simulink model "BFE_TestHarness"  (Simulink 8.6)
settings: Solver=FixedStepDiscrete  StartTime=0.0  StopTime=3  FixedStep=Ts  RelTol=1e-3
PreLoadFcn:
  | addpath('MBD_Tests')
  | 
  | load('Workspace\EnvVar.mat')
  | run('MBD_Tests\MBD_tests_init.m')
  | if exist('tl_preloadfcn','file'), tl_preloadfcn(gcs,402); end
PostLoadFcn:
  | if exist('tl_postloadfcn','file'), tl_postloadfcn(gcs,402); end
InitFcn:
  | if exist('tlds_init','file'), tlds_init(gcs); end
StartFcn:
  | if exist('tlds_start','file'), tlds_start(gcs); end
StopFcn:
  | if exist('tlds_stop','file'), tlds_stop(gcs); end
undefined symbols (not defined in the file): ddv, Ts, u2, u3, u4
libraries: tllib x11, simulink x8, LIB_TF_G_111 x2, LIB_TF_G_12_StepControl x2, LIB_TF_G_112 x1, LIB_TF_G_113 x1
(part 1 of 17)
PreSaveFcn:
  | if exist('tl_presavefcn','file'), tl_presavefcn(gcs); end
CloseFcn:
  | if exist('tl_closefcn','file'), tl_closefcn(gcs); end
settings Model: TL_MAIN_DATA={'codeopt',{'linebreaklimit',150,'cleancode',1},'logopt',{'mdlrefmode',2},'date',737167.70554642356,'codegenerationmode',2}  TLRevision=402  DS_PROJECTFILE=BFE_Data.dd  Creator=cedric.sauvage  LastModifiedBy=pierre-olivier.pilot
settings DataIOCC: MaxDataPoints=16000  SignalLoggingSaveFormat=Dataset
settings OptimizationCC: BlockReduction=off  OptimizeBlockIOStorage=off  BufferReuse=off  GlobalBufferReuse=off  ExpressionFolding=off  LocalBlockOutputs=off
settings DebuggingCC: CheckSSInitialOutputMsg=off  FcnCallInpInsideContextMsg=UseLocalSettings  BusObjectLabelMismatch=error  StrictBusMsg=ErrorOnBusTreatedAsVector  NonBusSignalsTreatedAsBus=error
settings HardwareCC: ProdHWDeviceType=Generic->Unspecified (assume 32-bit Generic)
settings ModelReferenceCC: ModelReferenceNumInstancesAllowed=Single

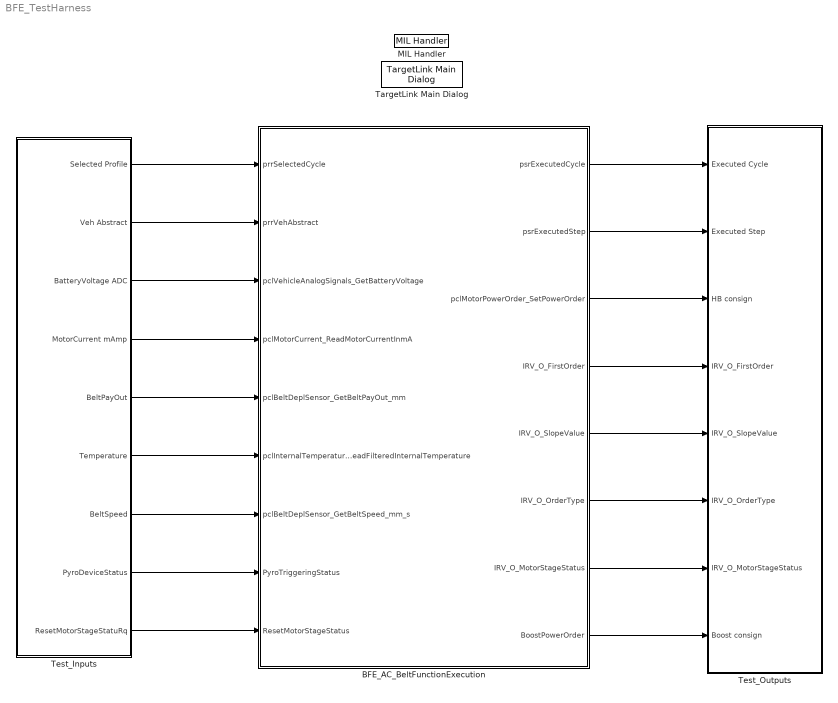
== system BFE_TestHarness ==
  BFE_AC_BeltFunctionExecution : Subsystem  Tag=TargetLink Simulation Frame  mask(TL_SimFrame){}
      settings: CopyFcn=if exist('tl_copyfcn','file'), tl_copyfcn(gcbh); end  NameChangeFcn=if exist('tl_framenamechangefcn','file'), tl_framenamechangefcn(gcbh); end
      settings: OpenFcn=|
      | if exist('open_tlsubsystem','file')
      |    open_tlsubsystem(gcbh);
      | else
      |    tlsubsystem = ...
      |       find_system(gcb, ...
      |       'LookUnderMasks','on', ...
      |       'FollowLinks','on', ...
      |       'Tag','MIL Subsystem');
      |    open_system(tlsubsystem);
      | end
      mask Display: disp('TargetLink\nModel-\nin-the-loop\nmode')
  MIL Handler : tllib/MIL Handler  data={'date',735951.66842159722}
  TargetLink Main Dialog : tllib/TargetLink Main Dialog  data=[]
  Test_Inputs : Subsystem
  Test_Outputs : Subsystem
  wires:
  Test_Inputs/2(Veh Abstract) -> BFE_AC_BeltFunctionExecution/2(prrVehAbstract)
  Test_Inputs/3(BatteryVoltage ADC) -> BFE_AC_BeltFunctionExecution/3(pclVehicleAnalogSignals_GetBatteryVoltage)
  Test_Inputs/4(MotorCurrent mAmp) -> BFE_AC_BeltFunctionExecution/4(pclMotorCurrent_ReadMotorCurrentInmA)
  Test_Inputs/5(BeltPayOut) -> BFE_AC_BeltFunctionExecution/5(pclBeltDeplSensor_GetBeltPayOut_mm)
  Test_Inputs/6(Temperature) -> BFE_AC_BeltFunctionExecution/6(pclInternalTemperature_ReadFilteredInternalTemperature)
  Test_Inputs/7(BeltSpeed) -> BFE_AC_BeltFunctionExecution/7(pclBeltDeplSensor_GetBeltSpeed_mm_s)
  Test_Inputs/1(Selected Profile) -> BFE_AC_BeltFunctionExecution/1(prrSelectedCycle)
  BFE_AC_BeltFunctionExecution/1(psrExecutedCycle) -> Test_Outputs/1(Executed Cycle)
  BFE_AC_BeltFunctionExecution/2(psrExecutedStep) -> Test_Outputs/2(Executed Step)
  BFE_AC_BeltFunctionExecution/3(pclMotorPowerOrder_SetPowerOrder) -> Test_Outputs/3(HB consign)
  Test_Inputs/8(PyroDeviceStatus) -> BFE_AC_BeltFunctionExecution/8(PyroTriggeringStatus)
  BFE_AC_BeltFunctionExecution/4(IRV_O_FirstOrder) -> Test_Outputs/4(IRV_O_FirstOrder)
  BFE_AC_BeltFunctionExecution/5(IRV_O_SlopeValue) -> Test_Outputs/5(IRV_O_SlopeValue)
  BFE_AC_BeltFunctionExecution/6(IRV_O_OrderType) -> Test_Outputs/6(IRV_O_OrderType)
  BFE_AC_BeltFunctionExecution/7(IRV_O_MotorStageStatus) -> Test_Outputs/7(IRV_O_MotorStageStatus)
  BFE_AC_BeltFunctionExecution/8(BoostPowerOrder) -> Test_Outputs/8(Boost consign)
  Test_Inputs/9(ResetMotorStageStatuRq) -> BFE_AC_BeltFunctionExecution/9(ResetMotorStageStatus)

== system BFE_TestHarness/BFE_AC_BeltFunctionExecution ==
  prrSelectedCycle : Inport
  prrVehAbstract : Inport  Port=2
  pclVehicleAnalogSignals_GetBatteryVoltage : Inport  Port=3
  pclMotorCurrent_ReadMotorCurrentInmA : Inport  Port=4
  pclBeltDeplSensor_GetBeltPayOut_mm : Inport  Port=5
  pclInternalTemperature_ReadFilteredInternalTemperature : Inport  Port=6
  pclBeltDeplSensor_GetBeltSpeed_mm_s : Inport  Port=7
  PyroTriggeringStatus : Inport  Port=8
  ResetMotorStageStatus : Inport  Port=9
  Subsystem : Subsystem  Tag=struct('sfcnName','BFE_AC_BeltFunctionExecution_sf','subFunction','','srcSubsystem','')  mask(TL_Enable){}
      settings: OpenFcn=warndlg(get_param(gcb,'MaskHelp'),'Serious Warning');
      mask Help: This subsystem keeps the TargetLink subsystem (subsystem with TargetLink blocks for production code generation), and is needed for the TargetLink simulation frame to work properly. DO NOT DELETE OR MODIFY IT!
  psrExecutedCycle : Outport
  psrExecutedStep : Outport  Port=2
  pclMotorPowerOrder_SetPowerOrder : Outport  Port=3
  IRV_O_FirstOrder : Outport  Port=4
  IRV_O_SlopeValue : Outport  Port=5
  IRV_O_OrderType : Outport  Port=6
  IRV_O_MotorStageStatus : Outport  Port=7
  BoostPowerOrder : Outport  Port=8
  wires:
  prrSelectedCycle/1 -> Subsystem/1(prrSelectedCycle)
  prrVehAbstract/1 -> Subsystem/2(prrVehAbstract)
  pclVehicleAnalogSignals_GetBatteryVoltage/1 -> Subsystem/3(pclVehicleAnalogSignals_GetBatteryVoltage)
  pclMotorCurrent_ReadMotorCurrentInmA/1 -> Subsystem/4(pclMotorCurrent_ReadMotorCurrentInmA)
  pclBeltDeplSensor_GetBeltPayOut_mm/1 -> Subsystem/5(pclBeltDeplSensor_GetBeltPayOut_mm)
  pclInternalTemperature_ReadFilteredInternalTemperature/1 -> Subsystem/6(pclInternalTemperature_ReadFilteredInternalTemperature)
  pclBeltDeplSensor_GetBeltSpeed_mm_s/1 -> Subsystem/7(pclBeltDeplSensor_GetBeltSpeed_mm_s)
  PyroTriggeringStatus/1 -> Subsystem/8(PyroTriggeringStatus)
  ResetMotorStageStatus/1 -> Subsystem/9(ResetMotorStageStatus)
  Subsystem/1(psrExecutedCycle) -> psrExecutedCycle/1
  Subsystem/2(psrExecutedStep) -> psrExecutedStep/1
  Subsystem/3(pclMotorPowerOrder_SetPowerOrder) -> pclMotorPowerOrder_SetPowerOrder/1
  Subsystem/4(IRV_O_FirstOrder) -> IRV_O_FirstOrder/1
  Subsystem/5(IRV_O_SlopeValue) -> IRV_O_SlopeValue/1
  Subsystem/6(IRV_O_OrderType) -> IRV_O_OrderType/1
  Subsystem/7(IRV_O_MotorStageStatus) -> IRV_O_MotorStageStatus/1
  Subsystem/8(BoostPowerOrder) -> BoostPowerOrder/1

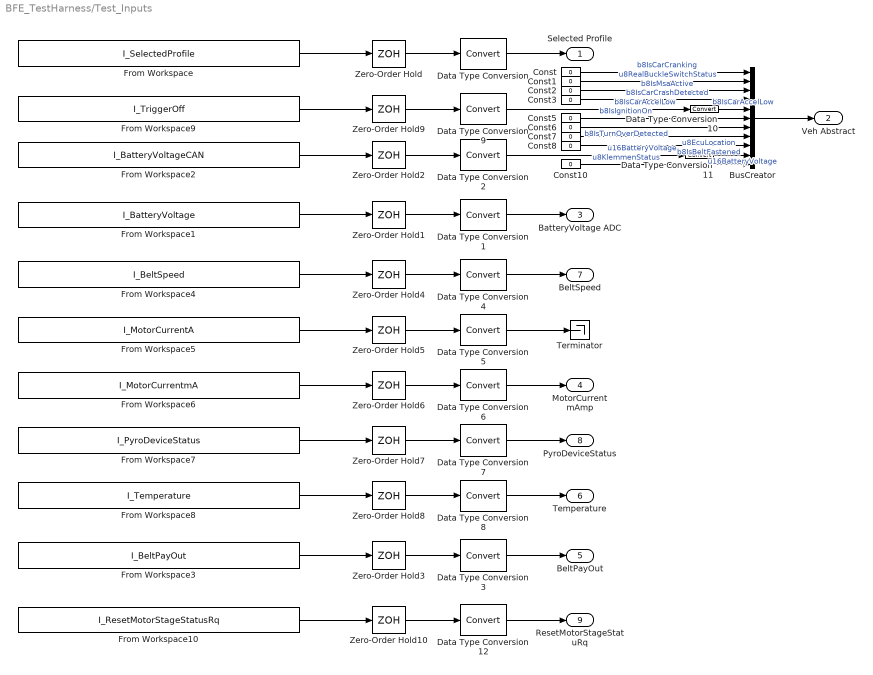
== system BFE_TestHarness/Test_Inputs ==
  BusCreator : BusCreator  Inputs=11
  Const{,1..3,5..8,10} (9 alike) : Constant  Value=0
  Data Type Conversion{,1..12} (13 alike) : DataTypeConversion
  From Workspace : FromWorkspace  VariableName=I_SelectedProfile  SampleTime=Ts  OutputAfterFinalValue=Holding final value
  From Workspace1 : FromWorkspace  VariableName=I_BatteryVoltage  SampleTime=Ts
  From Workspace10 : FromWorkspace  VariableName=I_ResetMotorStageStatusRq  SampleTime=Ts
  From Workspace2 : FromWorkspace  VariableName=I_BatteryVoltageCAN  SampleTime=Ts
  From Workspace3 : FromWorkspace  VariableName=I_BeltPayOut  SampleTime=Ts
  From Workspace4 : FromWorkspace  VariableName=I_BeltSpeed  SampleTime=Ts
  From Workspace5 : FromWorkspace  VariableName=I_MotorCurrentA  SampleTime=Ts
  From Workspace6 : FromWorkspace  VariableName=I_MotorCurrentmA  SampleTime=Ts
  From Workspace7 : FromWorkspace  VariableName=I_PyroDeviceStatus  SampleTime=Ts
  From Workspace8 : FromWorkspace  VariableName=I_Temperature  SampleTime=Ts
  From Workspace9 : FromWorkspace  VariableName=I_TriggerOff  SampleTime=Ts
  Terminator : Terminator
  Zero-Order Hold : ZeroOrderHold  SampleTime=-1
  Zero-Order Hold{1..10} (10 alike) : ZeroOrderHold  SampleTime=Ts
  Selected Profile : Outport
  Veh Abstract : Outport  Port=2
  BatteryVoltage ADC : Outport  Port=3
  MotorCurrent mAmp : Outport  Port=4
  BeltPayOut : Outport  Port=5
  Temperature : Outport  Port=6
  BeltSpeed : Outport  Port=7
  PyroDeviceStatus : Outport  Port=8
  ResetMotorStageStatuRq : Outport  Port=9
  wires:
  From Workspace/1 -> Zero-Order Hold/1
  Data Type Conversion/1 -> Selected Profile/1
  Zero-Order Hold1/1 -> Data Type Conversion1/1
  Data Type Conversion1/1 -> BatteryVoltage ADC/1
  Zero-Order Hold2/1 -> Data Type Conversion2/1
  Data Type Conversion2/1 -> Data Type Conversion11/1  "u16BatteryVoltage"
  Zero-Order Hold3/1 -> Data Type Conversion3/1
  Data Type Conversion3/1 -> BeltPayOut/1
  Zero-Order Hold4/1 -> Data Type Conversion4/1
  Data Type Conversion4/1 -> BeltSpeed/1
  Zero-Order Hold5/1 -> Data Type Conversion5/1
  Data Type Conversion5/1 -> Terminator/1
  Zero-Order Hold6/1 -> Data Type Conversion6/1
  Data Type Conversion6/1 -> MotorCurrent mAmp/1
  Zero-Order Hold7/1 -> Data Type Conversion7/1
  Data Type Conversion7/1 -> PyroDeviceStatus/1
  Zero-Order Hold8/1 -> Data Type Conversion8/1
  Data Type Conversion8/1 -> Temperature/1
  Zero-Order Hold9/1 -> Data Type Conversion9/1
  Data Type Conversion9/1 -> Data Type Conversion10/1  "b8IsCarAccelLow"
  From Workspace1/1 -> Zero-Order Hold1/1
  From Workspace2/1 -> Zero-Order Hold2/1
  From Workspace3/1 -> Zero-Order Hold3/1
  From Workspace4/1 -> Zero-Order Hold4/1
  From Workspace5/1 -> Zero-Order Hold5/1
  From Workspace6/1 -> Zero-Order Hold6/1
  From Workspace7/1 -> Zero-Order Hold7/1
  From Workspace8/1 -> Zero-Order Hold8/1
  From Workspace9/1 -> Zero-Order Hold9/1
  Const/1 -> BusCreator/1  "b8IsCarCranking"
  Const1/1 -> BusCreator/2  "u8RealBuckleSwitchStatus"
  Const2/1 -> BusCreator/3  "b8IsMsaActive"
  Const3/1 -> BusCreator/4  "b8IsCarCrashDetected"
  Const5/1 -> BusCreator/6  "b8IsIgnitionOn"
  Const6/1 -> BusCreator/7  "b8IsTurnOverDetected"
  Const7/1 -> BusCreator/8  "u8EcuLocation"
  Const8/1 -> BusCreator/9  "b8IsBeltFastened"
  Const10/1 -> BusCreator/11  "u8KlemmenStatus"
  Data Type Conversion10/1 -> BusCreator/5  "b8IsCarAccelLow"
  Data Type Conversion11/1 -> BusCreator/10  "u16BatteryVoltage"
  BusCreator/1 -> Veh Abstract/1
  Zero-Order Hold/1 -> Data Type Conversion/1
  Zero-Order Hold10/1 -> Data Type Conversion12/1
  Data Type Conversion12/1 -> ResetMotorStageStatuRq/1
  From Workspace10/1 -> Zero-Order Hold10/1

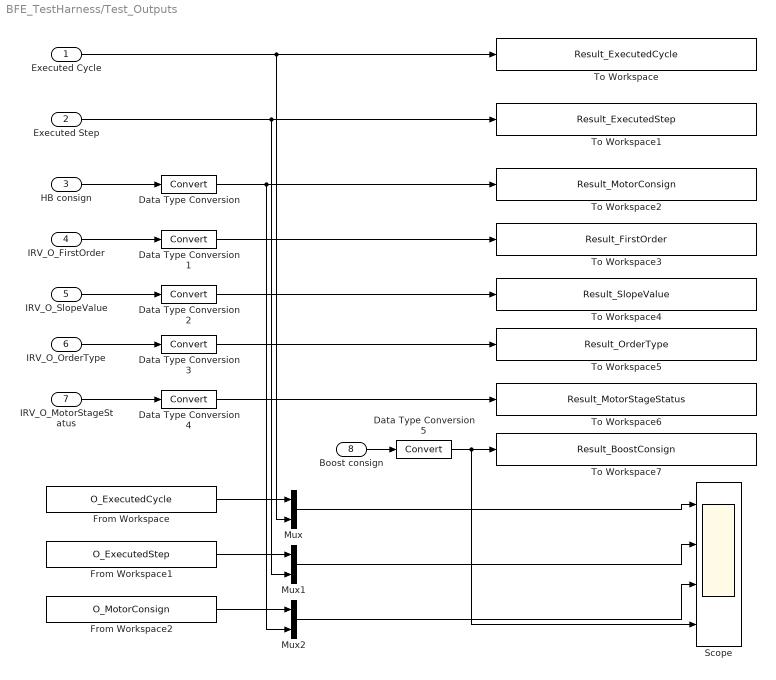
== system BFE_TestHarness/Test_Outputs ==
  Executed Cycle : Inport
  Executed Step : Inport  Port=2
  HB consign : Inport  Port=3
  IRV_O_FirstOrder : Inport  Port=4
  IRV_O_SlopeValue : Inport  Port=5
  IRV_O_OrderType : Inport  Port=6
  IRV_O_MotorStageStatus : Inport  Port=7
  Boost consign : Inport  Port=8
  Data Type Conversion{,1..5} (6 alike) : DataTypeConversion
  From Workspace : FromWorkspace  VariableName=O_ExecutedCycle  SampleTime=Ts
  From Workspace1 : FromWorkspace  VariableName=O_ExecutedStep  SampleTime=Ts
  From Workspace2 : FromWorkspace  VariableName=O_MotorConsign  SampleTime=Ts
  Mux : Mux  Inputs=2
  Mux1 : Mux  Inputs=2
  Mux2 : Mux  Inputs=2
  Scope : Scope  NumInputPorts=4
  To Workspace : ToWorkspace  VariableName=Result_ExecutedCycle  SaveFormat=Structure With Time  SampleTime=-1
  To Workspace1 : ToWorkspace  VariableName=Result_ExecutedStep  SaveFormat=Structure  SampleTime=-1
  To Workspace2 : ToWorkspace  VariableName=Result_MotorConsign  SaveFormat=Structure  SampleTime=-1
  To Workspace3 : ToWorkspace  VariableName=Result_FirstOrder  SaveFormat=Structure  SampleTime=-1
  To Workspace4 : ToWorkspace  VariableName=Result_SlopeValue  SaveFormat=Structure  SampleTime=-1
  To Workspace5 : ToWorkspace  VariableName=Result_OrderType  SaveFormat=Structure  SampleTime=-1
  To Workspace6 : ToWorkspace  VariableName=Result_MotorStageStatus  SaveFormat=Structure  SampleTime=-1
  To Workspace7 : ToWorkspace  VariableName=Result_BoostConsign  SaveFormat=Structure  SampleTime=-1
  wires:
  Executed Cycle/1 -> To Workspace/1, Mux/2
  Executed Step/1 -> To Workspace1/1, Mux1/2
  HB consign/1 -> Data Type Conversion/1
  Mux/1 -> Scope/1
  Mux1/1 -> Scope/2
  Mux2/1 -> Scope/3
  From Workspace/1 -> Mux/1
  From Workspace1/1 -> Mux1/1
  From Workspace2/1 -> Mux2/1
  Data Type Conversion/1 -> To Workspace2/1, Mux2/2
  IRV_O_FirstOrder/1 -> Data Type Conversion1/1
  IRV_O_SlopeValue/1 -> Data Type Conversion2/1
  IRV_O_OrderType/1 -> Data Type Conversion3/1
  Data Type Conversion1/1 -> To Workspace3/1
  Data Type Conversion2/1 -> To Workspace4/1
  Data Type Conversion3/1 -> To Workspace5/1
  IRV_O_MotorStageStatus/1 -> Data Type Conversion4/1
  Data Type Conversion4/1 -> To Workspace6/1
  Boost consign/1 -> Data Type Conversion5/1
  Data Type Conversion5/1 -> To Workspace7/1, Scope/4

== system BFE_TestHarness/BFE_AC_BeltFunctionExecution/Subsystem ==
  prrSelectedCycle : Inport
  prrVehAbstract : Inport  Port=2
  pclVehicleAnalogSignals_GetBatteryVoltage : Inport  Port=3
  pclMotorCurrent_ReadMotorCurrentInmA : Inport  Port=4
  pclBeltDeplSensor_GetBeltPayOut_mm : Inport  Port=5
  pclInternalTemperature_ReadFilteredInternalTemperature : Inport  Port=6
  pclBeltDeplSensor_GetBeltSpeed_mm_s : Inport  Port=7
  PyroTriggeringStatus : Inport  Port=8
  ResetMotorStageStatus : Inport  Port=9
  BFE_AC_BeltFunctionExecution : Subsystem  Tag=MIL Subsystem  Description=a  mask(MIL Subsystem){}
      settings: CopyFcn=if exist('tl_copyfcn','file'), tl_copyfcn(gcbh); end  NameChangeFcn=if exist('tl_namechangefcn','file'), tl_namechangefcn(gcbh); end  DestroyFcn=if exist('update_tl_main_dlg','file'), update_tl_main_dlg('TL_subs_display'); end
      mask Display: disp('TargetLink Subsystem')
  psrExecutedCycle : Outport
  psrExecutedStep : Outport  Port=2
  pclMotorPowerOrder_SetPowerOrder : Outport  Port=3
  IRV_O_FirstOrder : Outport  Port=4
  IRV_O_SlopeValue : Outport  Port=5
  IRV_O_OrderType : Outport  Port=6
  IRV_O_MotorStageStatus : Outport  Port=7
  BoostPowerOrder : Outport  Port=8
  wires:
  prrSelectedCycle/1 -> BFE_AC_BeltFunctionExecution/1(prrSelectedCycle)
  prrVehAbstract/1 -> BFE_AC_BeltFunctionExecution/2(prrVehAbstract)
  pclVehicleAnalogSignals_GetBatteryVoltage/1 -> BFE_AC_BeltFunctionExecution/3(pclVehicleAnalogSignals_GetBatteryVoltage)
  pclMotorCurrent_ReadMotorCurrentInmA/1 -> BFE_AC_BeltFunctionExecution/4(pclMotorCurrent_ReadMotorCurrentInmA)
  pclBeltDeplSensor_GetBeltPayOut_mm/1 -> BFE_AC_BeltFunctionExecution/5(pclBeltDeplSensor_GetBeltPayOut_mm)
  pclInternalTemperature_ReadFilteredInternalTemperature/1 -> BFE_AC_BeltFunctionExecution/6(pclInternalTemperature_ReadFilteredInternalTemperature)
  pclBeltDeplSensor_GetBeltSpeed_mm_s/1 -> BFE_AC_BeltFunctionExecution/7(pclBeltDeplSensor_GetBeltSpeed_mm_s)
  PyroTriggeringStatus/1 -> BFE_AC_BeltFunctionExecution/8(PyroTriggeringStatus)
  ResetMotorStageStatus/1 -> BFE_AC_BeltFunctionExecution/9(ResetMotorStageStatus)
  BFE_AC_BeltFunctionExecution/1(psrExecutedCycle) -> psrExecutedCycle/1
  BFE_AC_BeltFunctionExecution/2(psrExecutedStep) -> psrExecutedStep/1
  BFE_AC_BeltFunctionExecution/3(pclMotorPowerOrder_SetPowerOrder) -> pclMotorPowerOrder_SetPowerOrder/1
  BFE_AC_BeltFunctionExecution/4(IRV_O_FirstOrder) -> IRV_O_FirstOrder/1
  BFE_AC_BeltFunctionExecution/5(IRV_O_SlopeValue) -> IRV_O_SlopeValue/1
  BFE_AC_BeltFunctionExecution/6(IRV_O_OrderType) -> IRV_O_OrderType/1
  BFE_AC_BeltFunctionExecution/7(IRV_O_MotorStageStatus) -> IRV_O_MotorStageStatus/1
  BFE_AC_BeltFunctionExecution/8(BoostPowerOrder) -> BoostPowerOrder/1

== system BFE_TestHarness/BFE_AC_BeltFunctionExecution/Subsystem/BFE_AC_BeltFunctionExecution ==
  prrSelectedCycle : Inport
      settings: NameChangeFcn=if exist('tl_check_ports','file'), tl_check_ports(gcbh); end
      settings: CopyFcn=|
      | if exist('tl_reset_reviewflag','file')==2
      |     tl_reset_reviewflag(gcbh);
      | end
      | if exist('tl_check_ports','file')
      |     tl_check_ports(gcbh);
      | end
  prrVehAbstract : Inport  Port=2
      settings: NameChangeFcn=if exist('tl_check_ports','file'), tl_check_ports(gcbh); end
      settings: CopyFcn=|
      | if exist('tl_reset_reviewflag','file')==2
      |     tl_reset_reviewflag(gcbh);
      | end
      | if exist('tl_check_ports','file')
      |     tl_check_ports(gcbh);
      | end
  pclVehicleAnalogSignals_GetBatteryVoltage : Inport  Port=3
      settings: NameChangeFcn=if exist('tl_check_ports','file'), tl_check_ports(gcbh); end
      settings: CopyFcn=|
      | if exist('tl_reset_reviewflag','file')==2
      |     tl_reset_reviewflag(gcbh);
      | end
      | if exist('tl_check_ports','file')
      |     tl_check_ports(gcbh);
      | end
  pclMotorCurrent_ReadMotorCurrentInmA : Inport  Port=4
      settings: NameChangeFcn=if exist('tl_check_ports','file'), tl_check_ports(gcbh); end
      settings: CopyFcn=|
      | if exist('tl_reset_reviewflag','file')==2
      |     tl_reset_reviewflag(gcbh);
      | end
      | if exist('tl_check_ports','file')
      |     tl_check_ports(gcbh);
      | end
  pclBeltDeplSensor_GetBeltPayOut_mm : Inport  Port=5
      settings: NameChangeFcn=if exist('tl_check_ports','file'), tl_check_ports(gcbh); end
      settings: CopyFcn=|
      | if exist('tl_reset_reviewflag','file')==2
      |     tl_reset_reviewflag(gcbh);
      | end
      | if exist('tl_check_ports','file')
      |     tl_check_ports(gcbh);
      | end
  pclInternalTemperature_ReadFilteredInternalTemperature : Inport  Port=6
      settings: NameChangeFcn=if exist('tl_check_ports','file'), tl_check_ports(gcbh); end
      settings: CopyFcn=|
      | if exist('tl_reset_reviewflag','file')==2
      |     tl_reset_reviewflag(gcbh);
      | end
      | if exist('tl_check_ports','file')
      |     tl_check_ports(gcbh);
      | end
  pclBeltDeplSensor_GetBeltSpeed_mm_s : Inport  Port=7
      settings: NameChangeFcn=if exist('tl_check_ports','file'), tl_check_ports(gcbh); end
      settings: CopyFcn=|
      | if exist('tl_reset_reviewflag','file')==2
      |     tl_reset_reviewflag(gcbh);
      | end
      | if exist('tl_check_ports','file')
      |     tl_check_ports(gcbh);
      | end
  PyroTriggeringStatus : Inport  Port=8  mask(TL_Inport){data={'output',{'type','UInt8'},'date',735951.6686239352}}
      settings: DeleteFcn=if exist('delete_tlblock','file')==2,delete_tlblock(gcbh);end  OpenFcn=if exist('tl_open_blockdlg','file')==2,tl_open_blockdlg(gcbh);else,open_system(gcbh,'parameter');end
      settings: CopyFcn=|
      | if exist('tl_reset_reviewflag','file')==2
      |     tl_reset_reviewflag(gcbh);
      | end
      | if exist('tl_check_ports','file')
      |     tl_check_ports(gcbh);
      | end
      settings: NameChangeFcn=|
      | if exist('rename_tlblock','file')==2,rename_tlblock(gcbh);end
      | if exist('tl_check_ports','file'), tl_check_ports(gcbh); end
      mask Help: eval(['if exist(''tl_online_help'',''file'') == 2, tl_online_help(''Topic'',''TL_Inport''),else, web([''jar:file:///'',matlabroot,''/help/toolbox/simulink/help.jar!/slref/' lower(get_param(gcbh,'Blocktype')) '.html''], ''-helpbrowser''),end'])
      mask Display: plot([0.2 0.35 NaN 0.65 0.8],[0 1 NaN 0 1]);
  ResetMotorStageStatus : Inport  Port=9  mask(TL_Inport){data={'output',{'type','UInt8'},'date',735951.6686239352}}
      settings: DeleteFcn=if exist('delete_tlblock','file')==2,delete_tlblock(gcbh);end  OpenFcn=if exist('tl_open_blockdlg','file')==2,tl_open_blockdlg(gcbh);else,open_system(gcbh,'parameter');end
      settings: CopyFcn=|
      | if exist('tl_reset_reviewflag','file')==2
      |     tl_reset_reviewflag(gcbh);
      | end
      | if exist('tl_check_ports','file')
      |     tl_check_ports(gcbh);
      | end
      settings: NameChangeFcn=|
      | if exist('rename_tlblock','file')==2,rename_tlblock(gcbh);end
      | if exist('tl_check_ports','file'), tl_check_ports(gcbh); end
      mask Help: eval(['if exist(''tl_online_help'',''file'') == 2, tl_online_help(''Topic'',''TL_Inport''),else, web([''jar:file:///'',matlabroot,''/help/toolbox/simulink/help.jar!/slref/' lower(get_param(gcbh,'Blocktype')) '.html''], ''-helpbrowser''),end'])
      mask Display: plot([0.2 0.35 NaN 0.65 0.8],[0 1 NaN 0 1]);
  BFE_AC_BeltFunctionExecution : Subsystem
  psrExecutedCycle : Outport
      settings: NameChangeFcn=if exist('tl_check_ports','file'), tl_check_ports(gcbh); end
      settings: CopyFcn=|
      | if exist('tl_reset_reviewflag','file')==2
      |     tl_reset_reviewflag(gcbh);
      | end
      | if exist('tl_check_ports','file')
      |     tl_check_ports(gcbh);
      | end
  psrExecutedStep : Outport  Port=2
      settings: NameChangeFcn=if exist('tl_check_ports','file'), tl_check_ports(gcbh); end
      settings: CopyFcn=|
      | if exist('tl_reset_reviewflag','file')==2
      |     tl_reset_reviewflag(gcbh);
      | end
      | if exist('tl_check_ports','file')
      |     tl_check_ports(gcbh);
      | end
  pclMotorPowerOrder_SetPowerOrder : Outport  Port=3  mask(TL_Outport){data={'date',735951.66842629632}}
      settings: DeleteFcn=if exist('delete_tlblock','file')==2,delete_tlblock(gcbh);end  OpenFcn=if exist('tl_open_blockdlg','file')==2,tl_open_blockdlg(gcbh);else,open_system(gcbh,'parameter');end
      settings: CopyFcn=|
      | if exist('tl_reset_reviewflag','file')==2
      |     tl_reset_reviewflag(gcbh);
      | end
      | if exist('tl_check_ports','file')
      |     tl_check_ports(gcbh);
      | end
      settings: NameChangeFcn=|
      | if exist('rename_tlblock','file')==2,rename_tlblock(gcbh);end
      | if exist('tl_check_ports','file'), tl_check_ports(gcbh); end
      mask Help: eval(['if exist(''tl_online_help'',''file'') == 2, tl_online_help(''Topic'',''TL_Outport''),else, web([''jar:file:///'',matlabroot,''/help/toolbox/simulink/help.jar!/slref/' lower(get_param(gcbh,'Blocktype')) '.html''], ''-helpbrowser''),end'])
      mask Display: plot([0.2 0.35 NaN 0.65 0.8],[0 1 NaN 0 1]);
  IRV_O_FirstOrder : Outport  Port=4  mask(TL_Outport){data={'output',{'type','Int32'},'date',735951.66842549772}}
      settings: DeleteFcn=if exist('delete_tlblock','file')==2,delete_tlblock(gcbh);end  OpenFcn=if exist('tl_open_blockdlg','file')==2,tl_open_blockdlg(gcbh);else,open_system(gcbh,'parameter');end
      settings: CopyFcn=|
      | if exist('tl_reset_reviewflag','file')==2
      |     tl_reset_reviewflag(gcbh);
      | end
      | if exist('tl_check_ports','file')
      |     tl_check_ports(gcbh);
      | end
      settings: NameChangeFcn=|
      | if exist('rename_tlblock','file')==2,rename_tlblock(gcbh);end
      | if exist('tl_check_ports','file'), tl_check_ports(gcbh); end
      mask Help: eval(['if exist(''tl_online_help'',''file'') == 2, tl_online_help(''Topic'',''TL_Outport''),else, web([''jar:file:///'',matlabroot,''/help/toolbox/simulink/help.jar!/slref/' lower(get_param(gcbh,'Blocktype')) '.html''], ''-helpbrowser''),end'])
      mask Display: plot([0.2 0.35 NaN 0.65 0.8],[0 1 NaN 0 1]);
  IRV_O_SlopeValue : Outport  Port=5  mask(TL_Outport){data={'output',{'type','Int32'},'date',735951.66842468746}}
      settings: DeleteFcn=if exist('delete_tlblock','file')==2,delete_tlblock(gcbh);end  OpenFcn=if exist('tl_open_blockdlg','file')==2,tl_open_blockdlg(gcbh);else,open_system(gcbh,'parameter');end
      settings: CopyFcn=|
      | if exist('tl_reset_reviewflag','file')==2
      |     tl_reset_reviewflag(gcbh);
      | end
      | if exist('tl_check_ports','file')
      |     tl_check_ports(gcbh);
      | end
      settings: NameChangeFcn=|
      | if exist('rename_tlblock','file')==2,rename_tlblock(gcbh);end
      | if exist('tl_check_ports','file'), tl_check_ports(gcbh); end
      mask Help: eval(['if exist(''tl_online_help'',''file'') == 2, tl_online_help(''Topic'',''TL_Outport''),else, web([''jar:file:///'',matlabroot,''/help/toolbox/simulink/help.jar!/slref/' lower(get_param(gcbh,'Blocktype')) '.html''], ''-helpbrowser''),end'])
      mask Display: plot([0.2 0.35 NaN 0.65 0.8],[0 1 NaN 0 1]);
  IRV_O_OrderType : Outport  Port=6  mask(TL_Outport){data={'output',{'type','UInt8'},'date',735951.66842387733}}
      settings: DeleteFcn=if exist('delete_tlblock','file')==2,delete_tlblock(gcbh);end  OpenFcn=if exist('tl_open_blockdlg','file')==2,tl_open_blockdlg(gcbh);else,open_system(gcbh,'parameter');end
      settings: CopyFcn=|
      | if exist('tl_reset_reviewflag','file')==2
      |     tl_reset_reviewflag(gcbh);
      | end
      | if exist('tl_check_ports','file')
      |     tl_check_ports(gcbh);
      | end
      settings: NameChangeFcn=|
      | if exist('rename_tlblock','file')==2,rename_tlblock(gcbh);end
      | if exist('tl_check_ports','file'), tl_check_ports(gcbh); end
      mask Help: eval(['if exist(''tl_online_help'',''file'') == 2, tl_online_help(''Topic'',''TL_Outport''),else, web([''jar:file:///'',matlabroot,''/help/toolbox/simulink/help.jar!/slref/' lower(get_param(gcbh,'Blocktype')) '.html''], ''-helpbrowser''),end'])
      mask Display: plot([0.2 0.35 NaN 0.65 0.8],[0 1 NaN 0 1]);
  IRV_O_MotorStageStatus : Outport  Port=7  mask(TL_Outport){data={'output',{'type','UInt8'},'date',735951.66842307872}}
      settings: DeleteFcn=if exist('delete_tlblock','file')==2,delete_tlblock(gcbh);end  OpenFcn=if exist('tl_open_blockdlg','file')==2,tl_open_blockdlg(gcbh);else,open_system(gcbh,'parameter');end
      settings: CopyFcn=|
      | if exist('tl_reset_reviewflag','file')==2
      |     tl_reset_reviewflag(gcbh);
      | end
      | if exist('tl_check_ports','file')
      |     tl_check_ports(gcbh);
      | end
      settings: NameChangeFcn=|
      | if exist('rename_tlblock','file')==2,rename_tlblock(gcbh);end
      | if exist('tl_check_ports','file'), tl_check_ports(gcbh); end
      mask Help: eval(['if exist(''tl_online_help'',''file'') == 2, tl_online_help(''Topic'',''TL_Outport''),else, web([''jar:file:///'',matlabroot,''/help/toolbox/simulink/help.jar!/slref/' lower(get_param(gcbh,'Blocktype')) '.html''], ''-helpbrowser''),end'])
      mask Display: plot([0.2 0.35 NaN 0.65 0.8],[0 1 NaN 0 1]);
  BoostPowerOrder : Outport  Port=8  mask(TL_Outport){data={'date',735951.66842229164}}
      settings: DeleteFcn=if exist('delete_tlblock','file')==2,delete_tlblock(gcbh);end  OpenFcn=if exist('tl_open_blockdlg','file')==2,tl_open_blockdlg(gcbh);else,open_system(gcbh,'parameter');end
      settings: CopyFcn=|
      | if exist('tl_reset_reviewflag','file')==2
      |     tl_reset_reviewflag(gcbh);
      | end
      | if exist('tl_check_ports','file')
      |     tl_check_ports(gcbh);
      | end
      settings: NameChangeFcn=|
      | if exist('rename_tlblock','file')==2,rename_tlblock(gcbh);end
      | if exist('tl_check_ports','file'), tl_check_ports(gcbh); end
      mask Help: eval(['if exist(''tl_online_help'',''file'') == 2, tl_online_help(''Topic'',''TL_Outport''),else, web([''jar:file:///'',matlabroot,''/help/toolbox/simulink/help.jar!/slref/' lower(get_param(gcbh,'Blocktype')) '.html''], ''-helpbrowser''),end'])
      mask Display: plot([0.2 0.35 NaN 0.65 0.8],[0 1 NaN 0 1]);
  wires:
  prrSelectedCycle/1 -> BFE_AC_BeltFunctionExecution/1(prrSelectedCycle)
  prrVehAbstract/1 -> BFE_AC_BeltFunctionExecution/2(prrVehAbstract)
  pclVehicleAnalogSignals_GetBatteryVoltage/1 -> BFE_AC_BeltFunctionExecution/3(pclVehicleAnalogSignals_GetBatteryVoltage)
  pclMotorCurrent_ReadMotorCurrentInmA/1 -> BFE_AC_BeltFunctionExecution/4(pclMotorCurrent_ReadMotorCurrentInmA)
  pclBeltDeplSensor_GetBeltPayOut_mm/1 -> BFE_AC_BeltFunctionExecution/5(pclBeltDeplSensor_GetBeltPayOut_mm)
  pclInternalTemperature_ReadFilteredInternalTemperature/1 -> BFE_AC_BeltFunctionExecution/6(pclInternalTemperature_ReadFilteredInternalTemperature)
  pclBeltDeplSensor_GetBeltSpeed_mm_s/1 -> BFE_AC_BeltFunctionExecution/7(pclBeltDeplSensor_GetBeltSpeed_mm_s)
  BFE_AC_BeltFunctionExecution/1(psrExecutedCycle) -> psrExecutedCycle/1
  BFE_AC_BeltFunctionExecution/2(psrExecutedStep) -> psrExecutedStep/1
  BFE_AC_BeltFunctionExecution/3(pclMotorPowerOrder_SetPowerOrder) -> pclMotorPowerOrder_SetPowerOrder/1
  PyroTriggeringStatus/1 -> BFE_AC_BeltFunctionExecution/8(PyroTriggeringStatus)
  BFE_AC_BeltFunctionExecution/4(IRV_O_FirstOrder) -> IRV_O_FirstOrder/1
  BFE_AC_BeltFunctionExecution/5(IRV_O_SlopeValue) -> IRV_O_SlopeValue/1
  BFE_AC_BeltFunctionExecution/6(IRV_O_OrderType) -> IRV_O_OrderType/1
  BFE_AC_BeltFunctionExecution/7(IRV_O_MotorStageStatus) -> IRV_O_MotorStageStatus/1
  BFE_AC_BeltFunctionExecution/8(pclMotorPowerOrder_SetPowerOrder1) -> BoostPowerOrder/1
  ResetMotorStageStatus/1 -> BFE_AC_BeltFunctionExecution/9(ResetMotorStageStatus)

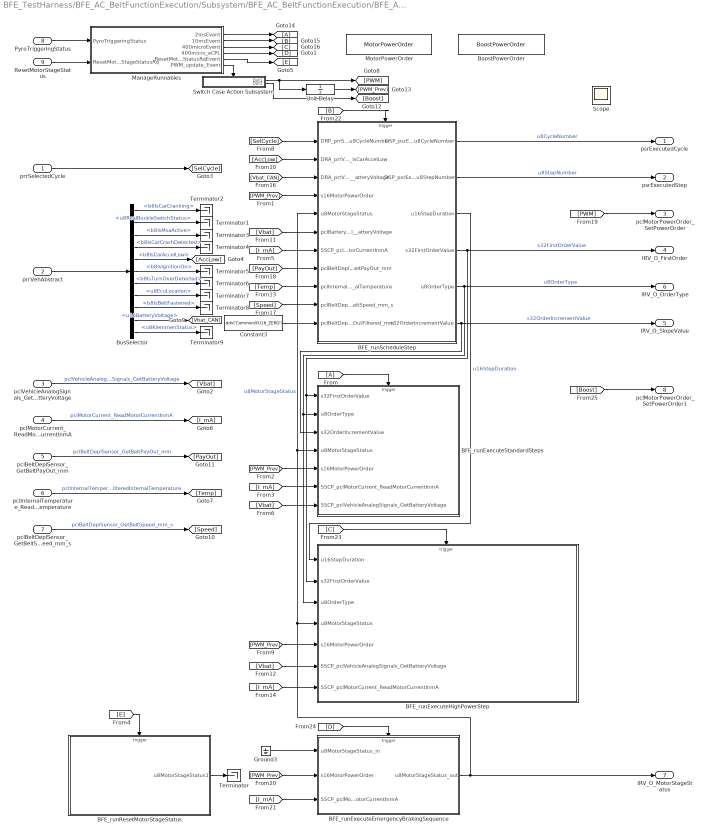
== system BFE_TestHarness/BFE_AC_BeltFunctionExecution/Subsystem/BFE_AC_BeltFunctionExecution/BFE_AC_BeltFunctionExecution ==
  prrSelectedCycle : Inport
  prrVehAbstract : Inport  Port=2
  pclVehicleAnalogSignals_GetBatteryVoltage : Inport  Port=3
  pclMotorCurrent_ReadMotorCurrentInmA : Inport  Port=4
  pclBeltDeplSensor_GetBeltPayOut_mm : Inport  Port=5
  pclInternalTemperature_ReadFilteredInternalTemperature : Inport  Port=6
  pclBeltDeplSensor_GetBeltSpeed_mm_s : Inport  Port=7
  PyroTriggeringStatus : Inport  Port=8
  ResetMotorStageStatus : Inport  Port=9
  BFE_runExecuteEmergencyBrakingSequence : Subsystem  TreatAsAtomicUnit=on
  BFE_runExecuteHighPowerStep : Subsystem  TreatAsAtomicUnit=on
  BFE_runExecuteStandardSteps : Subsystem  TreatAsAtomicUnit=on
  BFE_runResetMotorStageStatus : Subsystem  TreatAsAtomicUnit=on
  BFE_runScheduleStep : Subsystem  TreatAsAtomicUnit=on
  BoostPowerOrder : DataStoreMemory  RequirementInfo={} %GIDa_a27f5205_5aa0_4fe0_9bfb_d5ffa7252d0a  DataStoreName=BoostPowerOrder  WriteAfterWriteMsg=warning  WriteAfterReadMsg=warning  OutDataTypeStr=int16  mask(TL_DataStoreMemory){data={'output',{'variable','BFE/BoostPowerOrder'},'autoscaling',{'mode',2},'date',735951.66845049767}}
      settings: CopyFcn=if exist('tl_reset_reviewflag','file')==2,tl_reset_reviewflag(gcbh);end  DeleteFcn=if exist('delete_tlblock','file')==2,delete_tlblock(gcbh);end  NameChangeFcn=if exist('rename_tlblock','file')==2,rename_tlblock(gcbh);end  OpenFcn=if exist('tl_open_blockdlg','file')==2,tl_open_blockdlg(gcbh);else,open_system(gcbh,'parameter');end
      mask Help: eval(['if exist(''tl_online_help'',''file'') == 2, tl_online_help(''Topic'',''TL_DataStoreMemory''),else, web([''jar:file:///'',matlabroot,''/help/toolbox/simulink/help.jar!/slref/' lower(get_param(gcbh,'Blocktype')) '.html''], ''-helpbrowser''),end'])
      mask Display: plot([-0.05, 1.05, NaN, -0.05, 1.05],[.01, .01, NaN, .99, .99])
  BusSelector : BusSelector  OutputSignals=b8IsCarCranking,u8RealBuckleSwitchStatus,b8IsMsaActive,b8IsCarCrashDetected,b8IsCarAccelLow,b8IsIgnitionOn,b8IsTurnOverDetected,u8EcuLocation,b8IsBeltFastened,u16BatteryVoltage,u8KlemmenStatus
  Constant3 : Constant  RequirementInfo={} %GIDa_9fc74ee4_2a33_4b48_aaae_58408e10ad1d  Value=ddv('Common/KU16_ZERO')  OutDataTypeStr=uint16  mask(TL_Constant){data={'output',{'variable','Common/KU16_ZERO'},'autoscaling',{'mode',2,'scalingvalid',1},'date',735951.66845013888}}
      settings: CopyFcn=if exist('tl_reset_reviewflag','file')==2,tl_reset_reviewflag(gcbh);end  DeleteFcn=if exist('delete_tlblock','file')==2,delete_tlblock(gcbh);end  NameChangeFcn=if exist('rename_tlblock','file')==2,rename_tlblock(gcbh);end  OpenFcn=if exist('tl_open_blockdlg','file')==2,tl_open_blockdlg(gcbh);else,open_system(gcbh,'parameter');end
      mask Help: eval(['if exist(''tl_online_help'',''file'') == 2, tl_online_help(''Topic'',''TL_Constant''),else, web([''jar:file:///'',matlabroot,''/help/toolbox/simulink/help.jar!/slref/' lower(get_param(gcbh,'Blocktype')) '.html''], ''-helpbrowser''),end'])
      mask Display: plot([-0.05, 1.05, NaN, -0.05, 1.05],[.01, .01, NaN, .99, .99])
  Ground3 : Ground
  ManageRunnables : Subsystem  RequirementInfo={} %GIDa_eb8f3858_a721_4fb6_8c8c_9100dbc0a282
  MotorPowerOrder : DataStoreMemory  RequirementInfo={} %GIDa_2ca9386b_2301_41eb_b156_3c7fc8d332f8  DataStoreName=MotorPowerOrder  WriteAfterWriteMsg=warning  WriteAfterReadMsg=warning  OutDataTypeStr=int16  mask(TL_DataStoreMemory){data={'output',{'variable','BFE/MotorPowerOrder'},'autoscaling',{'mode',2},'date',735951.66842833336}}
      settings: CopyFcn=if exist('tl_reset_reviewflag','file')==2,tl_reset_reviewflag(gcbh);end  DeleteFcn=if exist('delete_tlblock','file')==2,delete_tlblock(gcbh);end  NameChangeFcn=if exist('rename_tlblock','file')==2,rename_tlblock(gcbh);end  OpenFcn=if exist('tl_open_blockdlg','file')==2,tl_open_blockdlg(gcbh);else,open_system(gcbh,'parameter');end
      mask Help: eval(['if exist(''tl_online_help'',''file'') == 2, tl_online_help(''Topic'',''TL_DataStoreMemory''),else, web([''jar:file:///'',matlabroot,''/help/toolbox/simulink/help.jar!/slref/' lower(get_param(gcbh,'Blocktype')) '.html''], ''-helpbrowser''),end'])
      mask Display: plot([-0.05, 1.05, NaN, -0.05, 1.05],[.01, .01, NaN, .99, .99])
  Scope : Scope
  Switch Case Action Subsystem : Subsystem  RequirementInfo={} %GIDa_23231537_58f7_4f9a_af00_3ee5c94bcfd0  TreatAsAtomicUnit=on
  Terminator{,1..9} (10 alike) : Terminator
      Terminator1 settings: RequirementInfo={} %GIDa_a6acd51e_31f7_4016_8236_67519406a53f
      Terminator2 settings: RequirementInfo={} %GIDa_23bcebab_55a3_4e04_baae_8085a8f9b643
      Terminator3 settings: RequirementInfo={} %GIDa_f3640e03_a634_4f1a_ba7c_ca00bb4a731a
      Terminator4 settings: RequirementInfo={} %GIDa_df0fd7b9_011d_460b_84fa_aca799d44bbd
      Terminator5 settings: RequirementInfo={} %GIDa_f2d55dce_61fe_492f_aa84_6b71d0034c74
      Terminator6 settings: RequirementInfo={} %GIDa_5243533d_6e74_4bf2_a2fd_c72045971767
      Terminator7 settings: RequirementInfo={} %GIDa_58312b2b_125e_408f_bfe0_440c0347e4f9
      Terminator8 settings: RequirementInfo={} %GIDa_d88e7c9d_2b22_4f2c_bb3a_a7d55f1ed99a
      Terminator9 settings: RequirementInfo={} %GIDa_e1c463e4_3f74_4358_8c1d_0f95b41680cf
  Unit Delay : UnitDelay  RequirementInfo={} %GIDa_a17179d9_6bb4_4eff_b007_e36b3b5e0945  SampleTime=-1  mask(TL_UnitDelay){data={'date',735951.66842682869}}
      settings: CopyFcn=if exist('tl_reset_reviewflag','file')==2,tl_reset_reviewflag(gcbh);end  DeleteFcn=if exist('delete_tlblock','file')==2,delete_tlblock(gcbh);end  NameChangeFcn=if exist('rename_tlblock','file')==2,rename_tlblock(gcbh);end  OpenFcn=if exist('tl_open_blockdlg','file')==2,tl_open_blockdlg(gcbh);else,open_system(gcbh,'parameter');end
      mask Help: eval(['if exist(''tl_online_help'',''file'') == 2, tl_online_help(''Topic'',''TL_UnitDelay''),else, web([''jar:file:///'',matlabroot,''/help/toolbox/simulink/help.jar!/slref/' lower(get_param(gcbh,'Blocktype')) '.html''], ''-helpbrowser''),end'])
      mask Display: plot([-0.05, 1.05, NaN, -0.05, 1.05],[.01, .01, NaN, .99, .99])
  psrExecutedCycle : Outport
  psrExecutedStep : Outport  Port=2
  pclMotorPowerOrder_SetPowerOrder : Outport  Port=3
  IRV_O_FirstOrder : Outport  Port=4
  IRV_O_SlopeValue : Outport  Port=5
  IRV_O_OrderType : Outport  Port=6
  IRV_O_MotorStageStatus : Outport  Port=7
  pclMotorPowerOrder_SetPowerOrder1 : Outport  Port=8
  wires:
  prrVehAbstract/1 -> BusSelector/1
  BFE_runScheduleStep/1(DSP_psrExecut__u8CycleNumber) -> psrExecutedCycle/1  "u8CycleNumber"
  BFE_runScheduleStep/2(DSP_psrExecut___u8StepNumber) -> psrExecutedStep/1  "u8StepNumber"
  BusSelector/1 -> Terminator2/1  "<b8IsCarCranking>"
  BusSelector/2 -> Terminator1/1  "<u8RealBuckleSwitchStatus>"
  BusSelector/3 -> Terminator3/1  "<b8IsMsaActive>"
  BusSelector/4 -> Terminator4/1  "<b8IsCarCrashDetected>"
  BusSelector/6 -> Terminator5/1  "<b8IsIgnitionOn>"
  BusSelector/7 -> Terminator6/1  "<b8IsTurnOverDetected>"
  BusSelector/8 -> Terminator7/1  "<u8EcuLocation>"
  BusSelector/9 -> Terminator8/1  "<b8IsBeltFastened>"
  BusSelector/11 -> Terminator9/1  "<u8KlemmenStatus>"
  prrSelectedCycle/1 -> [SelCycle]
  BusSelector/5 -> [AccLow]  "<b8IsCarAccelLow>"
  BusSelector/10 -> [Vbat_CAN]  "<u16BatteryVoltage>"
  pclVehicleAnalogSignals_GetBatteryVoltage/1 -> [Vbat]  "pclVehicleAnalogSignals_GetBatteryVoltage"
  pclMotorCurrent_ReadMotorCurrentInmA/1 -> [I_mA]  "pclMotorCurrent_ReadMotorCurrentInmA"
  pclInternalTemperature_ReadFilteredInternalTemperature/1 -> [Temp]  "pclInternalTemperature_ReadFilteredInternalTemperature"
  pclBeltDeplSensor_GetBeltSpeed_mm_s/1 -> [Speed]  "pclBeltDeplSensor_GetBeltSpeed_mm_s"
  pclBeltDeplSensor_GetBeltPayOut_mm/1 -> [PayOut]  "pclBeltDeplSensor_GetBeltPayOut_mm"
  Switch Case Action Subsystem/1(Out1) -> [PWM], Unit Delay/1
  Unit Delay/1 -> [PWM_Prev]
  ManageRunnables/1(2msEvent) -> [A]
  ManageRunnables/2(10msEvent) -> [B]
  ManageRunnables/6(PWM_update_Event) -> Switch Case Action Subsystem/Trigger
  ManageRunnables/3(400microEvent) -> [C]
  [PWM] -> pclMotorPowerOrder_SetPowerOrder/1
  [AccLow] -> BFE_runScheduleStep/2(DRA_prrVehAbs__IsCarAccelLow)
  [SelCycle] -> BFE_runScheduleStep/1(DRP_prrSelect__u8CycleNumber)
  [Vbat_CAN] -> BFE_runScheduleStep/3(DRA_prrVehAbs__atteryVoltage)
  [PWM_Prev] -> BFE_runScheduleStep/4(s16MotorPowerOrder)
  [Vbat] -> BFE_runScheduleStep/6(pclBatteryVol__atteryVoltage)
  [I_mA] -> BFE_runScheduleStep/7(SSCP_pclMotorCurrent_ReadMotorCurrentInmA)
  [PayOut] -> BFE_runScheduleStep/8(pclBeltDeplSe__BeltPayOut_mm)
  [Temp] -> BFE_runScheduleStep/9(pclInternalTe__alTemperature)
  [Speed] -> BFE_runScheduleStep/10(pclBeltDeplSe__eltSpeed_mm_s)
  [I_mA] -> BFE_runExecuteStandardSteps/6(SSCP_pclMotorCurrent_ReadMotorCurrentInmA)
  [Vbat] -> BFE_runExecuteStandardSteps/7(SSCP_pclVehicleAnalogSignals_GetBatteryVoltage)
  [PWM_Prev] -> BFE_runExecuteHighPowerStep/5(s16MotorPowerOrder)
  [Vbat] -> BFE_runExecuteHighPowerStep/6(SSCP_pclVehicleAnalogSignals_GetBatteryVoltage)
  [I_mA] -> BFE_runExecuteHighPowerStep/7(SSCP_pclMotorCurrent_ReadMotorCurrentInmA)
  Ground3/1 -> BFE_runExecuteEmergencyBrakingSequence/1(u8MotorStageStatus_in)
  [PWM_Prev] -> BFE_runExecuteEmergencyBrakingSequence/2(s16MotorPowerOrder)
  [I_mA] -> BFE_runExecuteEmergencyBrakingSequence/3(SSCP_pclMotorCurrent_ReadMotorCurrentInmA)
  BFE_runScheduleStep/3(u16StepDuration) -> BFE_runExecuteHighPowerStep/1(u16StepDuration)  "u16StepDuration"
  BFE_runScheduleStep/5(u8OrderType) -> BFE_runExecuteHighPowerStep/3(u8OrderType), BFE_runExecuteStandardSteps/2(u8OrderType), IRV_O_OrderType/1  "u8OrderType"
  BFE_runExecuteEmergencyBrakingSequence/1(u8MotorStageStatus_out) -> IRV_O_MotorStageStatus/1, BFE_runScheduleStep/5(u8MotorStageStatus), BFE_runExecuteStandardSteps/4(u8MotorStageStatus), BFE_runExecuteHighPowerStep/4(u8MotorStageStatus)  "u8MotorStageStatus"
  [PWM_Prev] -> BFE_runExecuteStandardSteps/5(s16MotorPowerOrder)
  BFE_runScheduleStep/4(s32FirstOrderValue) -> BFE_runExecuteHighPowerStep/2(s32FirstOrderValue), BFE_runExecuteStandardSteps/1(s32FirstOrderValue), IRV_O_FirstOrder/1  "s32FirstOrderValue"
  [B] -> BFE_runScheduleStep/Trigger
  [A] -> BFE_runExecuteStandardSteps/Trigger
  [C] -> BFE_runExecuteHighPowerStep/Trigger
  ManageRunnables/4(400micro_eCPL) -> [D]
  [D] -> BFE_runExecuteEmergencyBrakingSequence/Trigger
  BFE_runScheduleStep/6(s32OrderIncrementValue) -> BFE_runExecuteStandardSteps/3(s32OrderIncrementValue), IRV_O_SlopeValue/1  "s32OrderIncrementValue"
  PyroTriggeringStatus/1 -> ManageRunnables/1(PyroTriggeringStatus)
  Switch Case Action Subsystem/2(Out2) -> [Boost]
  [Boost] -> pclMotorPowerOrder_SetPowerOrder1/1
  Constant3/1 -> BFE_runScheduleStep/11(pclBeltDeplSe__BeltPayOutFiltered_mm)
  BFE_runResetMotorStageStatus/1(u8MotorStageStatus1) -> Terminator/1
  ManageRunnables/5(ResetMotorStageStatusRqEvent) -> [E]
  [E] -> BFE_runResetMotorStageStatus/Trigger
  ResetMotorStageStatus/1 -> ManageRunnables/2(ResetMotorStageStatusRq)
